simulink model "transformer3windings"  (R2018a)
settings: Solver=VariableStepAuto  StartTime=0.0  StopTime=0.1  RelTol=1e-4
values from neighbouring files (symbols this model uses):
  ang = 0.7    [transformer2wind.m]    (also in transformer3wind.m)
  Freq = 60    [Autotransformer.m]    (also in transformer2wind.m; transformer3wind.m)
  K12 = 240/2400    (= 0.1)    [transformer3wind.m]
  K13 = K12    (= 0.1)    [transformer3wind.m]
  L1 = 0.92/(2*pi*Freq)    (= 0.00244037579408)    [Autotransformer.m]    (also in transformer2wind.m = 0.00119366207319; transformer3wind.m = 0.00119366207319)
  L2 = 0.009/(2*pi*Freq)    (= 2.38732414638e-05)    [Autotransformer.m]    (also in transformer2wind.m = 1.19366207319e-05; transformer3wind.m = 1.19366207319e-05)
  L3 = 0.0045/(2*pi*Freq)    (= 1.19366207319e-05)    [transformer3wind.m]
  Ll2 = Xl2/(2*pi*Freq)    (= 0.000305080078488)    [transformer3wind.m]
  Ll3 = Ll2    (= 0.000305080078488)    [transformer3wind.m]
  Lo = 4370/(2*pi*Freq)    (= 11.5917850219)    [Autotransformer.m]    (also in transformer2wind.m = 4.11150269654; transformer3wind.m = 4.11150269654)
  R1 = 0.72    [Autotransformer.m]    (also in transformer2wind.m = 0.2; transformer3wind.m = 0.2)
  R2 = 0.007    [Autotransformer.m]    (also in transformer2wind.m = 0.002; transformer3wind.m = 0.002)
  R3 = 0.002    [transformer3wind.m]
  Rl2 = 0.5*120109.7/(625*625)    (= 0.153740416)    [transformer3wind.m]
  Rl3 = Rl2    (= 0.153740416)    [transformer3wind.m]
  Ro = 632    [Autotransformer.m]    (also in transformer2wind.m = 10000; transformer3wind.m = 10000)
  S = 50000    [Autotransformer.m]    (also in transformer2wind.m = 150000; transformer3wind.m = 150000)
  V1 = 2400    [Autotransformer.m]    (also in transformer3wind.m)
  V2 = 240    [Autotransformer.m]    (also in transformer2wind.m; transformer3wind.m)
  V3 = 240    [transformer3wind.m]
  Vs = 2405*sqrt(2)    [Autotransformer.m]    (also in transformer2wind.m = 2455*sqrt(2); transformer3wind.m = 2455*sqrt(2))
libraries: powerlib x13
settings Model: Creator=Noor  LastModifiedBy=Noor

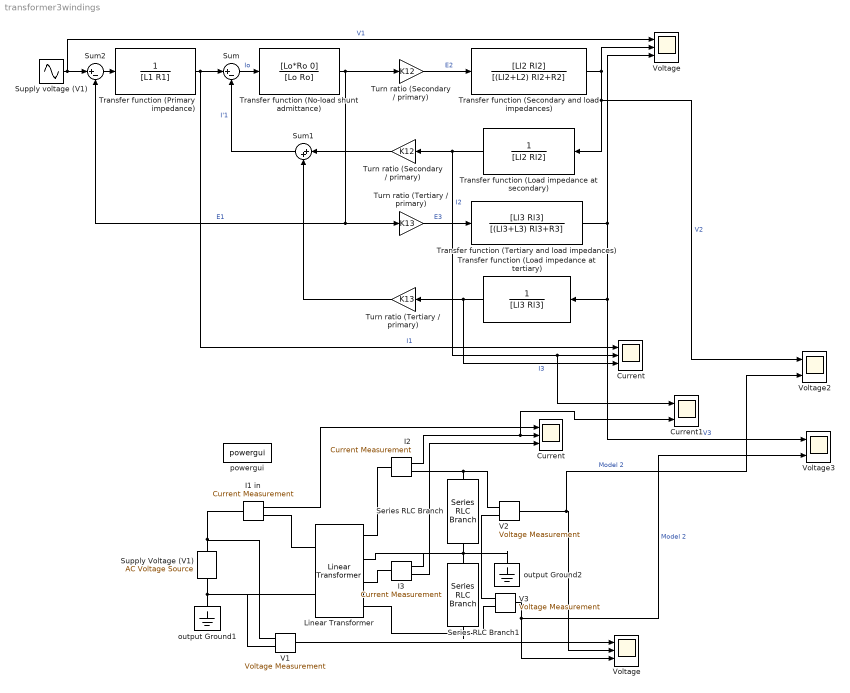
== system transformer3windings ==
  " Voltage" : Scope  NumInputPorts=3
  " Voltage2" : Scope  NumInputPorts=2
  Current : Scope  NumInputPorts=3
  "Current " : Scope  NumInputPorts=3
  Current1 : Scope  NumInputPorts=2
  I1 in : powerlib/Measurements/Current Measurement  Tag=PoWeRsYsTeMmEaSuReMeNt  PhasorSimulation=off  OutputType=Magnitude  PSBequivalent=0
  "I2 " : powerlib/Measurements/Current Measurement  Tag=PoWeRsYsTeMmEaSuReMeNt  PhasorSimulation=off  OutputType=Magnitude  PSBequivalent=0
  "I3 " : powerlib/Measurements/Current Measurement  Tag=PoWeRsYsTeMmEaSuReMeNt  PhasorSimulation=off  OutputType=Magnitude  PSBequivalent=0
  Linear Transformer : powerlib/Elements/Linear Transformer  UNITS=SI  NominalPower=[S Freq]  winding1=[V1 R1 L1]  winding2=[V2 R2 L3]  ThreeWindings=on  winding3=[V3 R3 L3]  RmLm=[Ro Lo]  Measurements=None  DataType=on
  Series RLC Branch : powerlib/Elements/Series RLC Branch  LConnTagsString=__new0  RConnTagsString=__new0  BranchType=RL  Resistance=Rl2  Inductance=Ll2  SetiL0=off  InitialCurrent=0  Capacitance=1e-6  Setx0=off  InitialVoltage=0  Measurements=None
  Series RLC Branch1 : powerlib/Elements/Series RLC Branch  LConnTagsString=__new0  RConnTagsString=__new0  BranchType=RL  Resistance=Rl3  Inductance=Ll3  SetiL0=off  InitialCurrent=0  Capacitance=1e-6  Setx0=off  InitialVoltage=0  Measurements=None
  Sum : Sum  Inputs=|+-
  Sum1 : Sum  Inputs=|++
  Sum2 : Sum  Inputs=|+-
  Supply Voltage (V1) : powerlib/Electrical Sources/AC Voltage Source  Description=source block  Amplitude=Vs  Phase=ang  Frequency=Freq  SampleTime=0  Measurements=None  BusType=swing  Pref=10e3  Qref=0  Qmin=-inf  Qmax=+inf
      settings: AttributesFormatString=\n
  Supply voltage (V1) : Sin  Amplitude=Vs  Frequency=2*pi*Freq  Phase=ang*pi/180  SampleTime=0
  Transfer function (Load impedance at secondary) : TransferFcn  Denominator=[Ll2 Rl2]
  Transfer function (Load impedance at tertiary) : TransferFcn  Denominator=[Ll3 Rl3]
  Transfer function (No-load shunt admittance) : TransferFcn  Numerator=[Lo*Ro 0]  Denominator=[Lo Ro]
  Transfer function (Primary impedance) : TransferFcn  Denominator=[L1 R1]
  Transfer function (Secondary and load impedances) : TransferFcn  Numerator=[Ll2 Rl2]  Denominator=[(Ll2+L2) Rl2+R2]
  Transfer function (Tertiary and load impedances) : TransferFcn  Numerator=[Ll3 Rl3]  Denominator=[(Ll3+L3) Rl3+R3]
  Turn ratio (Secondary / primary) : Gain  Gain=K12
  "Turn ratio (Secondary / primary) " : Gain  Gain=K12
  Turn ratio (Tertiary / primary) : Gain  Gain=K13
  "Turn ratio (Tertiary / primary) " : Gain  Gain=K13
  V1 : powerlib/Measurements/Voltage Measurement  Tag=PoWeRsYsTeMmEaSuReMeNt  PhasorSimulation=off  OutputType=Magnitude  PSBequivalent=0
  V2 : powerlib/Measurements/Voltage Measurement  Tag=PoWeRsYsTeMmEaSuReMeNt  PhasorSimulation=off  OutputType=Magnitude  PSBequivalent=0
  V3 : powerlib/Measurements/Voltage Measurement  Tag=PoWeRsYsTeMmEaSuReMeNt  PhasorSimulation=off  OutputType=Magnitude  PSBequivalent=0
  "Voltage " : Scope  NumInputPorts=3
  Voltage3 : Scope  NumInputPorts=2
  output Ground1 : powerlib/Elements/Ground  LConnTagsString=a
  output Ground2 : powerlib/Elements/Ground  LConnTagsString=a
  powergui : powerlib/powergui  SimulationMode=Continuous  SampleTime=0  frequency=60  Iterations=50  frequencyindice=60  Pbase=100e6  ErrMax=1e-4  UnitsV=kV  UnitsW=MW  buscounter=0  FunctionMessages=off  echomessages=off  EnableUseOfTLC=off  CurrentSourceSwitches=off  DisableSnubberDevices=off  DisableRonSwitches=off  DisableVfSwitches=off  DisplayEquations=off  SolverType=Tustin/Backward Euler (TBE)  Interpol=off  ExternalGateDelay=off  methode=off  Ts=100  x0status=blocks  SPID=off  SwTol=0  HookPort=off  RestoreLinks=warning  ResistiveCurrentMeasurement=off  Frange=[0:2:500]  Ylog=off  Xlog=on  ShowGrid=off  save=off  variable=ZData  structure=0  ZoomFFT=on  StartTime=0.0  cycles=1  DisplayStyle=1  fundamental=60  FreqAxis=off  MaxFrequency=1000  frequencyindicesteady=1  RmsSteady=1  display=off
  wires:
  Supply voltage (V1)/1 -> " Voltage"/1, Sum2/1  "V1"
  Sum/1 -> Transfer function (No-load shunt admittance)/1  "Io"
  Transfer function (No-load shunt admittance)/1 -> Turn ratio (Secondary / primary)/1, Turn ratio (Tertiary / primary)/1, Sum2/2  "E1"
  Sum2/1 -> Transfer function (Primary impedance)/1
  I1 in/1 -> "Current "/1
  Transfer function (Primary impedance)/1 -> Sum/1, Current/1  "I1"
  Sum1/1 -> Sum/2  "I'1"
  Transfer function (Secondary and load impedances)/1 -> " Voltage"/2, " Voltage2"/1, Transfer function (Load impedance at secondary)/1  "V2"
  Transfer function (Load impedance at secondary)/1 -> "Turn ratio (Secondary / primary) "/1, Current1/1, Current/2  "I2"
  Transfer function (Load impedance at tertiary)/1 -> "Turn ratio (Tertiary / primary) "/1, Current/3  "I3"
  Transfer function (Tertiary and load impedances)/1 -> Voltage3/1, Transfer function (Load impedance at tertiary)/1, " Voltage"/3  "V3"
  Turn ratio (Secondary / primary)/1 -> Transfer function (Secondary and load impedances)/1  "E2"
  Turn ratio (Tertiary / primary)/1 -> Transfer function (Tertiary and load impedances)/1  "E3"
  "Turn ratio (Secondary / primary) "/1 -> Sum1/1
  "Turn ratio (Tertiary / primary) "/1 -> Sum1/2
  "I2 "/1 -> Current1/2, "Current "/2
  "I3 "/1 -> "Current "/3
  V1/1 -> "Voltage "/1
  V2/1 -> " Voltage2"/2, "Voltage "/2  "Model 2"
  V3/1 -> Voltage3/2, "Voltage "/3  "Model 2"
  connections:
  Series RLC Branch/RConn1 -- V2/LConn2 -- V3/LConn1 -- output Ground2/LConn1 -- Linear Transformer/RConn2 -- "I3 "/RConn1 -- Series RLC Branch1/LConn1
  "I2 "/RConn1 -- V2/LConn1 -- Series RLC Branch/LConn1
  Linear Transformer/LConn1 -- I1 in/RConn1
  Supply Voltage (V1)/RConn1 -- I1 in/LConn1 -- V1/LConn1
  output Ground1/LConn1 -- V1/LConn2 -- Linear Transformer/LConn2 -- Supply Voltage (V1)/LConn1
  Series RLC Branch1/RConn1 -- Linear Transformer/RConn4 -- V3/LConn2
  "I2 "/LConn1 -- Linear Transformer/RConn1
  "I3 "/LConn1 -- Linear Transformer/RConn3
